simulink model "GoldenModel"  (R2024b)
settings: Solver=VariableStepAuto  StartTime=0.0  StopTime=10e-3  RelTol=1e-3
libraries: dspvision x5, dspsrcs4 x3, commchan3 x1, dspsnks4 x1
settings Model: Creator=mykola  LastModifiedBy=mykola

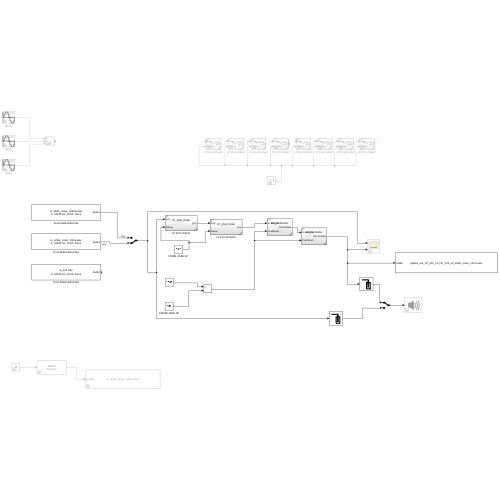
[thumbnail: Simulink's stored preview of the top-level diagram]
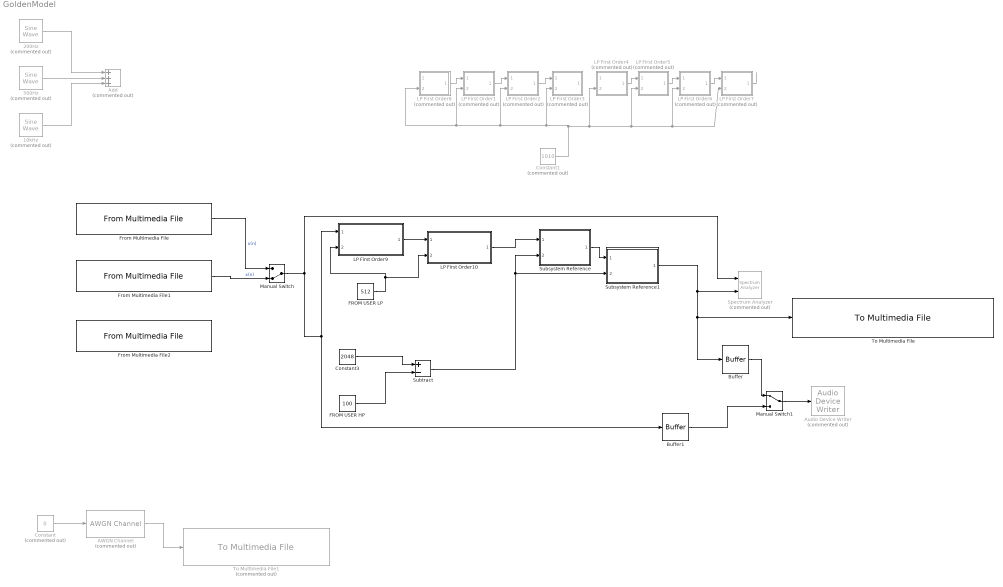
== system GoldenModel ==
  10kHz : dspsrcs4/Sine Wave  Commented=on  Amplitude=0.3  Frequency=10e3  Phase=0  SampleMode=Discrete  OutComplex=Real  CompMethod=Trigonometric fcn  TableSize=Speed  SampleTime=1/44100  SamplesPerFrame=1  ResetState=Restart at time zero  OutputFrames=off  dataType=double  wordLen=16  udDataType=sfix(16)  fracBitsMode=Best precision  numFracBits=15  OutDataTypeStr=double  LastOutDataTypeStr=double
  200Hz : dspsrcs4/Sine Wave  Commented=on  Amplitude=0.3  Frequency=200  Phase=0  SampleMode=Discrete  OutComplex=Real  CompMethod=Trigonometric fcn  TableSize=Speed  SampleTime=1/44100  SamplesPerFrame=1  ResetState=Restart at time zero  OutputFrames=off  dataType=double  wordLen=16  udDataType=sfix(16)  fracBitsMode=Best precision  numFracBits=15  OutDataTypeStr=double  LastOutDataTypeStr=double
  500Hz : dspsrcs4/Sine Wave  Commented=on  Amplitude=0.3  Frequency=500  Phase=0  SampleMode=Discrete  OutComplex=Real  CompMethod=Trigonometric fcn  TableSize=Speed  SampleTime=1/44100  SamplesPerFrame=1  ResetState=Restart at time zero  OutputFrames=off  dataType=double  wordLen=16  udDataType=sfix(16)  fracBitsMode=Best precision  numFracBits=15  OutDataTypeStr=double  LastOutDataTypeStr=double
  AWGN Channel : commchan3/AWGN Channel  Commented=on  LegacyMode=off  NoiseMethod="Signal to noise ratio  (SNR)"  noiseMode="Signal to noise ratio  (SNR)"  EbNo=10  EsNo=10  SNR=0  BitsPerSymbol=1  SignalPower=1  SamplesPerSymbol=1  SymbolPeriod=1  VarianceSource=Parameter  Variance=1  RandomStream=Global stream  Seed=67  SimulateUsing=Code generation
  Add : Sum  Commented=on  Inputs=+++
  Audio Device Writer : dspsnks4/Audio Device Writer  Commented=on  Driver=ALSA  Device=Default  InheritSampleRate=on  SampleRate=44100  BitDepth=16-bit integer  BufferSize=4096  NumBuffers=10  DefaultOutputChannelMapping=on  OutputChannelMapping=1:2  OutputNumUnderrunSamples=off  DriverIdx=8  DeviceWarnFlag=''
  Buffer : Buffer  N=512  OutputFrames=off
  Buffer1 : Buffer  N=512  OutputFrames=off
  Constant : Constant  Commented=on  Value=0  SampleTime=1/44100
  Constant1 : Constant  Commented=on  Value=1010
  Constant3 : Constant  Value=2048
  FROM USER HP : Constant  Value=100
  FROM USER LP : Constant  Value=512
  From Multimedia File : dspvision/From Multimedia File  inputFilename=/home/mykola/eda/designs/AudioASIC/audio_test/in_white_noise_100ms.wav  readRange=[1 Inf]  loop=on  numPlays=inf  outputStreams=Audio only  videoDataType=single  audioDataType=double  inheritSampleTime=on  userDefinedSampleTime=1/30  noAudioOutput=off  isIntensityVideo=off  fourcc=RGB  colorVideoFormat=One multidimensional signal  outputEOF=off  dataOrg=Column-major  audioFrameSize=1  computeAudioFrameSize=off  outSamplingMode=Sample based
      settings: LibrarySourceBlock=dspsrcs4/From Multimedia File
  From Multimedia File1 : dspvision/From Multimedia File  inputFilename=/home/mykola/eda/designs/AudioASIC/audio_test/in_white_noise_10ms.wav  readRange=[1 Inf]  loop=on  numPlays=inf  outputStreams=Audio only  videoDataType=single  audioDataType=double  inheritSampleTime=on  userDefinedSampleTime=1/30  noAudioOutput=off  isIntensityVideo=off  fourcc=RGB  colorVideoFormat=One multidimensional signal  outputEOF=off  dataOrg=Column-major  audioFrameSize=1  computeAudioFrameSize=off  outSamplingMode=Sample based
      settings: LibrarySourceBlock=dspsrcs4/From Multimedia File
  From Multimedia File2 : dspvision/From Multimedia File  inputFilename=/home/mykola/eda/designs/AudioASIC/audio_test/in_10s.wav  readRange=[1 Inf]  loop=on  numPlays=inf  outputStreams=Audio only  videoDataType=single  audioDataType=double  inheritSampleTime=on  userDefinedSampleTime=1/30  noAudioOutput=off  isIntensityVideo=off  fourcc=RGB  colorVideoFormat=One multidimensional signal  outputEOF=off  dataOrg=Column-major  audioFrameSize=1  computeAudioFrameSize=off  outSamplingMode=Sample based
      settings: LibrarySourceBlock=dspsrcs4/From Multimedia File
  LP First Order{1..8} (8 alike) : Subsystem  Commented=on  ReferencedSubsystem=LP_First_Order
  LP First Order10 : Subsystem  ReferencedSubsystem=LP_First_Order
  LP First Order9 : Subsystem  ReferencedSubsystem=LP_First_Order
  Manual Switch : ManualSwitch  CurrentSetting=0
  Manual Switch1 : ManualSwitch
  Spectrum Analyzer : SpectrumAnalyzer  Commented=on  NumInputPorts=2  WindowPosition=[1385.000000,172.000000,1096.000000,758.000000,]  Visible=on  ScopeFrameLocation=window  PlotAsTwoSidedSpectrum=off  WindowInvariantSamplesPerUpdate=on  YLimits=[-118.68408256,27.77349841]  ShowLegend=on
  Subsystem Reference : Subsystem  ReferencedSubsystem=HP_FirstOrder
  Subsystem Reference1 : Subsystem  ReferencedSubsystem=HP_FirstOrder
  Subtract : Sum  Inputs=+-
  To Multimedia File : dspvision/To Multimedia File  outputFilename=/home/mykola/eda/designs/AudioASIC/audio_test/golden_out_LP_512_x2_HP_100_x2_white_noise_10ms.wav  streamSelection=Audio only  videoCompressor=None (uncompressed)  audioCompressor=None (uncompressed)  imagePorts=One multidimensional signal  fileType=WAV  audioDatatype=16-bit integer  fourcc=RGB  audioBitRate=128  audioQuality=75  videoQuality=75  mj2000CompFactor=10
      settings: LibrarySourceBlock=dspsnks4/To Multimedia File
  To Multimedia File1 : dspvision/To Multimedia File  Commented=on  outputFilename=/home/mykola/eda/designs/AudioASIC/audio_test/in_white_noise_100ms.wav  streamSelection=Audio only  videoCompressor=None (uncompressed)  audioCompressor=None (uncompressed)  imagePorts=One multidimensional signal  fileType=WAV  audioDatatype=16-bit integer  fourcc=RGB  audioBitRate=128  audioQuality=75  videoQuality=75  mj2000CompFactor=10
      settings: LibrarySourceBlock=dspsnks4/To Multimedia File
  wires:
  AWGN Channel/1 -> To Multimedia File1/1
  Constant/1 -> AWGN Channel/1
  200Hz/1 -> Add/1
  500Hz/1 -> Add/2
  10kHz/1 -> Add/3
  From Multimedia File/1 -> Manual Switch/1  "x(n)"
  From Multimedia File1/1 -> Manual Switch/2  "x(n)"
  LP First Order6/1 -> LP First Order7/1
  LP First Order5/1 -> LP First Order6/1
  LP First Order4/1 -> LP First Order5/1
  LP First Order2/1 -> LP First Order3/1
  LP First Order1/1 -> LP First Order2/1
  LP First Order8/1 -> LP First Order1/1
  LP First Order7/1 -> ?
  Constant1/1 -> LP First Order7/2, LP First Order6/2, LP First Order5/2, LP First Order4/2, LP First Order3/2, LP First Order2/2, LP First Order1/2, LP First Order8/2
  Subsystem Reference1/1 -> Buffer/1, To Multimedia File/1, Spectrum Analyzer/2
  Buffer/1 -> Manual Switch1/1
  Manual Switch/1 -> LP First Order9/1, Buffer1/1, Spectrum Analyzer/1
  Manual Switch1/1 -> Audio Device Writer/1
  Buffer1/1 -> Manual Switch1/2
  Constant3/1 -> Subtract/1
  FROM USER HP/1 -> Subtract/2
  Subtract/1 -> Subsystem Reference1/2, Subsystem Reference/2
  Subsystem Reference/1 -> Subsystem Reference1/1
  FROM USER LP/1 -> LP First Order10/2, LP First Order9/2
  LP First Order9/1 -> LP First Order10/1
  LP First Order10/1 -> Subsystem Reference/1
